simulink model "BPSK"  (Simulink 6.1)
settings: Solver=ode45  StartTime=0.0  StopTime=1  RelTol=1e-3
libraries: commdigbbndpm2 x2, commchan2 x1, commrandsrc2 x1, commsink2 x1
settings Model: LastModifiedBy=Administrator  StrictBusMsg=Warning
settings OptimizationCC: InlineInvariantSignals=off

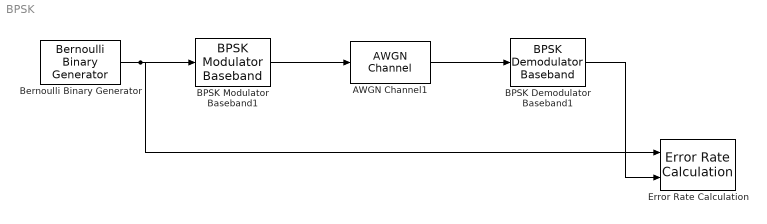
== system BPSK ==
  AWGN Channel1 : commchan2/AWGN Channel  seed=67  noiseMode="Signal to noise ratio  (Eb/No)"  EbNodB=ebn0  EsNodB=10  SNRdB=10  bitsPerSym=1  Ps=1  Tsym=1e-6  variance=1
  BPSK Demodulator Baseband1 : commdigbbndpm2/BPSK Demodulator Baseband  Ph=0  numSamp=1
  BPSK Modulator Baseband1 : commdigbbndpm2/BPSK Modulator Baseband  Ph=0  numSamp=1
  Bernoulli Binary Generator : commrandsrc2/Bernoulli Binary Generator  P=0.5  seed=66  Ts=1e-6  frameBased=on  sampPerFrame=10  orient=off
  Error Rate Calculation : commsink2/Error Rate Calculation  N=0  st_delay=0  cp_mode=Entire frame  subframe=[]  PMode=Workspace  WsName=ErrorVec  RsMode2=off  stop=off  numErr=100  maxBits=1e6
  wires:
  Bernoulli Binary Generator/1 -> Error Rate Calculation/1, BPSK Modulator Baseband1/1
  BPSK Demodulator Baseband1/1 -> Error Rate Calculation/2
  AWGN Channel1/1 -> BPSK Demodulator Baseband1/1
  BPSK Modulator Baseband1/1 -> AWGN Channel1/1
